simulink model "ScriptDemo"  (R2022b)
settings: configuration reference "TmVcThermal_Configuration_sub" (kept outside this file)
undefined symbols (not defined in the file): aaaa, bbbb, cTmComprCtrl_D_u8HvacFlowTable_db, cTmComprCtrl_D_u8HvacFlowTable_sw, cTmComprCtrl_n_i16ChillCmpIMax, cTmComprCtrl_n_i16ChillCmpIMin, cTmComprCtrl_n_i16ChillCmpIMin666, cTmComprCtrl_n_i16ChillCmpPMax, cTmComprCtrl_n_i16ChillCmpPMin, cTmComprCtrl_n_i16CmpChillCoolRpmKiMax, cTmComprCtrl_n_i16CmpChillCoolRpmKiMin, cTmComprCtrl_n_i16CmpChillCoolRpmKpMax, cTmComprCtrl_n_i16CmpChillCoolRpmKpMin, cTmComprCtrl_n_i16CmpCoolRpmKiMax, cTmComprCtrl_n_i16CmpCoolRpmKiMin, cTmComprCtrl_n_i16CmpCoolRpmKpMax, cTmComprCtrl_n_i16CmpCoolRpmKpMin, cTmComprCtrl_n_i16SM4CmpHeatKiMax, cTmComprCtrl_n_i16SM4CmpHeatKiMin, cTmComprCtrl_n_i16SM4CmpHeatKpMax, cTmComprCtrl_n_i16SM4CmpHeatKpMin, cTmComprCtrl_n_i16SM5CmpHeatKiMax, cTmComprCtrl_n_i16SM5CmpHeatKiMin, cTmComprCtrl_n_i16SM5CmpHeatKpMax, cTmComprCtrl_n_i16SM5CmpHeatKpMin, cTmComprCtrl_n_i16SM6CmpHeatKiMax, cTmComprCtrl_n_i16SM6CmpHeatKiMin, cTmComprCtrl_n_i16SM6CmpHeatKpMax, cTmComprCtrl_n_i16SM6CmpHeatKpMin, cTmComprCtrl_n_u16CmpMaxSpdFanFltLimt, cTmComprCtrl_n_u16CmpMaxSpdLoSidePFltLimt, cTmComprCtrl_n_u16CmpMaxSpdSensorFltLimt, cTmComprCtrl_n_u16CompMinRpm, cTmComprCtrl_n_u16CompRpmIncThres, cTmComprCtrl_t_u16BattCooltFFPeriod, cTmComprCtrl_t_u16BattCooltPIPeriod, cTmComprCtrl_t_u16CmpCoolFFPeriod, cTmComprCtrl_t_u16CmpCoolPIPeriod, cTmComprCtrl_t_u16CoolCmpChillFFPeriod, cTmComprCtrl_t_u16CoolCmpChillPIPeriod, cTmComprCtrl_t_u16SM4CmpHeatFFPeriod, cTmComprCtrl_t_u16SM4CmpHeatPIPeriod, cTmComprCtrl_t_u16SM5CmpHeatFFPeriod, cTmComprCtrl_t_u16SM5CmpHeatPIPeriod, cTmComprCtrl_t_u16SM6CmpHeatFFPeriod, cTmComprCtrl_t_u16SM6CmpHeatPIPeriod, cTmComprCtrl_Te_EvapClearInteg, cTmComprCtrl_Te_i16HpReqTempSaturoffset, cTmComprCtrl_Te_i16SatLpReplaceDiff, cTmComprCtrl_Te_i16SM3BatDiffStartEvapDecOffset, cTmComprCtrl_Te_i16SM3EvapLo, cTmComprCtrl_Te_i16SM3TBatDiffEntEvapDecOffset, cTmComprCtrl_Te_i16SM3TBatDiffEntEvapDecOffsetQuit, cTmComprCtrl_Te_s32ErrCmpChillPIContinueCoolH, cTmComprCtrl_Te_s32ErrCmpChillPIContinueCoolL, cTmComprCtrl_Te_s32ErrCmpPIContinueChillH, cTmComprCtrl_Te_s32ErrCmpPIContinueChillL, cTmComprCtrl_Te_s32ErrCmpPIContinueCoolH, cTmComprCtrl_Te_s32ErrCmpPIContinueCoolL, cTmComprCtrl_Te_s32ErrCmpPIContinueHeatH ... (+398)
libraries: simulink x782, PCMULib x640, simulink_need_slupdate x4
(part 15 of 41)

== system ScriptDemo/Create/createMerge/Before/SM6 ==
  note: 制热cycle的时候，水回路功能模式为12
  sTmSigProces_Te_s32HeatrAirTReqRamp : Inport  OutDataTypeStr=single
  sTmSigProces_Te_s32HvacHexAirTFilter : Inport  Port=2  OutDataTypeStr=single
  sTmSigProces_Te_s32TempInlet : Inport  Port=3  OutDataTypeStr=single
  sTmSigProces_Te_s32SatHp : Inport  Port=4  OutDataTypeStr=single
  sTmComprCtrl_D_u8HvacFlowLevel : Inport  Port=5  OutDataTypeStr=uint8
  xTmComprCtrl_B_CompOnReqCompOn : Inport  Port=6  OutDataTypeStr=boolean
  yTmHvchCtrl_B_HpcPtcEnad : Inport  Port=7  OutDataTypeStr=boolean
  yTmRefriModeMgr_B_HeatModeInCycle : Inport  Port=8  OutDataTypeStr=boolean
  Action Port : ActionPort
  Constant : Constant  Value=cTmComprCtrl_n_i16SM6CmpHeatKpMax  OutDataTypeStr=int16
  Constant15 : Constant  Value=cTmComprCtrl_Te_s32ErrCmpPIContinueHeatL  OutDataTypeStr=single
  Constant16 : Constant  Value=cTmComprCtrl_n_i16SM6CmpHeatKiMin  OutDataTypeStr=int16
  Constant18 : Constant  Value=cTmComprCtrl_n_i16SM6CmpHeatKiMax  OutDataTypeStr=int16
  Constant2 : Constant  Value=cTmComprCtrl_n_u16CompMinRpm
  Constant7 : Constant  Value=cTmComprCtrl_t_u16SM6CmpHeatPIPeriod  OutDataTypeStr=uint16
  Constant8 : Constant  Value=cTmComprCtrl_n_i16SM6CmpHeatKpMin  OutDataTypeStr=int16
  Constant9 : Constant  Value=cTmComprCtrl_Te_s32ErrCmpPIContinueHeatH  OutDataTypeStr=single
  ID26282_SM6FF : Subsystem
  ID26284_SM6Error : Subsystem
  Logical Operator : Logic  Operator=NOT  AllPortsSameDT=off  OutDataTypeStr=boolean
  SM6FFEnable : Subsystem
  SM6_Ki : Subsystem
  SM6_Kp : Subsystem
  rSM6_n_u16DisOverrideValue : Outport  OutDataTypeStr=uint16
  rSM6_t_u16PIPeriod : Outport  Port=2  OutDataTypeStr=uint16
  rSM6_Te_s32UpErrStop : Outport  Port=3  OutDataTypeStr=single
  rSM6_n_u16ComprRpmFF : Outport  Port=4  OutDataTypeStr=uint16
  rSM6_n_u16ComprRpmKp : Outport  Port=5  OutDataTypeStr=uint16
  rSM6_Te_s32LowErrStop : Outport  Port=6  OutDataTypeStr=single
  rSM6_n_i16KpUpLimit : Outport  Port=7  OutDataTypeStr=int16
  rSM6_n_i16KpLowLimit : Outport  Port=8  OutDataTypeStr=int16
  rSM6_n_i16KiUpLimit : Outport  Port=9  OutDataTypeStr=int16
  rSM6_n_i16KiLowLimit : Outport  Port=10  OutDataTypeStr=int16
  xSM6_B_Enable : Outport  Port=11  OutDataTypeStr=boolean
  rSM6_n_u16ComprRpmKi : Outport  Port=12  OutDataTypeStr=uint16
  rSM6_Te_s32TempError : Outport  Port=13  OutDataTypeStr=single
  wires:
  ID26284_SM6Error/1(rTmComprCtrl_Te_s32TempError) -> [rTmComprCtrl_Te_s32TempError]
  [sTmComprCtrl_D_u8HvacFlowLevel] -> ID26282_SM6FF/1(sTmComprCtrl_D_u8HvacFlowLevel)
  [sTmSigProces_Te_s32TempInlet] -> ID26282_SM6FF/2(sTmSigProces_Te_s32TempInlet)
  [sTmSigProces_Te_s32HeatrAirTReqRamp] -> ID26282_SM6FF/3(sTmSigProces_Te_s32HeatrAirTReqRamp)
  [sTmComprCtrl_D_u8HvacFlowLevel] -> SM6_Ki/1(sTmComprCtrl_D_u8HvacFlowLevel)
  [sTmSigProces_Te_s32TempInlet] -> SM6_Ki/2(sTmSigProces_Te_s32TempInlet)
  [rTmComprCtrl_Te_s32TempError] -> SM6_Ki/3(rTmComprCtrl_Te_s32TempError)
  [sTmComprCtrl_D_u8HvacFlowLevel] -> SM6_Kp/1(sTmComprCtrl_D_u8HvacFlowLevel)
  [sTmSigProces_Te_s32TempInlet] -> SM6_Kp/2(sTmSigProces_Te_s32TempInlet)
  [rTmComprCtrl_Te_s32TempError] -> SM6_Kp/3(rTmComprCtrl_Te_s32TempError)
  [sTmSigProces_Te_s32SatHp] -> ID26284_SM6Error/1(sTmSigProces_Te_s32SatHp)
  [yTmHvchCtrl_B_HpcPtcEnad] -> ID26284_SM6Error/2(yTmHvchCtrl_B_HpcPtcEnad)
  [sTmSigProces_Te_s32HeatrAirTReqRamp] -> ID26284_SM6Error/3(sTmSigProces_Te_s32HeatrAirTReqRamp)
  [sTmSigProces_Te_s32HvacHexAirTFilter] -> ID26284_SM6Error/4(sTmSigProces_Te_s32HvacHexAirTFilter)
  sTmSigProces_Te_s32HeatrAirTReqRamp/1 -> [sTmSigProces_Te_s32HeatrAirTReqRamp]
  sTmSigProces_Te_s32HvacHexAirTFilter/1 -> [sTmSigProces_Te_s32HvacHexAirTFilter]
  sTmSigProces_Te_s32TempInlet/1 -> [sTmSigProces_Te_s32TempInlet]
  sTmSigProces_Te_s32SatHp/1 -> [sTmSigProces_Te_s32SatHp]
  sTmComprCtrl_D_u8HvacFlowLevel/1 -> [sTmComprCtrl_D_u8HvacFlowLevel]
  xTmComprCtrl_B_CompOnReqCompOn/1 -> [xTmComprCtrl_B_CompOnReqCompOn]
  yTmHvchCtrl_B_HpcPtcEnad/1 -> [yTmHvchCtrl_B_HpcPtcEnad]
  ID26282_SM6FF/1(SM6FF) -> [rTmComprCtrl_n_u16ComprRpmFF]
  SM6_Ki/1(SM6Ki) -> [rTmComprCtrl_n_u16ComprRpmKi]
  SM6_Kp/1(SM6Kp) -> [rTmComprCtrl_n_u16ComprRpmKp]
  SM6FFEnable/1(SM6FFEnable_B_SM6FFEnable) -> [SM6FFEnable_B_SM6FFEnable]
  [xTmComprCtrl_B_CompOnReqCompOn] -> SM6FFEnable/1(xTmComprCtrl_B_CompOnReqCompOn)
  [SM6FFEnable_B_SM6FFEnable] -> ID26282_SM6FF/Enable
  Constant/1 -> [rTmComprCtrl_n_i16KpUpLimit]
  Constant2/1 -> [rTmComprCtrl_n_u16DisOverrideValue]
  Constant9/1 -> [rTmComprCtrl_Te_s32UpErrStop]
  Constant8/1 -> [rTmComprCtrl_n_i16KpLowLimit]
  Constant15/1 -> [rTmComprCtrl_Te_s32LowErrStop]
  Constant7/1 -> [rTmComprCtrl_t_u16PIPeriod]
  Constant16/1 -> [rTmComprCtrl_n_i16KiLowLimit]
  Logical Operator/1 -> [xTmComprCtrl_B_Enable]
  Constant18/1 -> [rTmComprCtrl_n_i16KiUpLimit]
  [yTmRefriModeMgr_B_HeatModeInCycle] -> Logical Operator/1
  yTmRefriModeMgr_B_HeatModeInCycle/1 -> [yTmRefriModeMgr_B_HeatModeInCycle]
  [rTmComprCtrl_n_u16DisOverrideValue] -> rSM6_n_u16DisOverrideValue/1
  [rTmComprCtrl_t_u16PIPeriod] -> rSM6_t_u16PIPeriod/1
  [rTmComprCtrl_Te_s32UpErrStop] -> rSM6_Te_s32UpErrStop/1
  [rTmComprCtrl_n_u16ComprRpmFF] -> rSM6_n_u16ComprRpmFF/1
  [rTmComprCtrl_n_u16ComprRpmKp] -> rSM6_n_u16ComprRpmKp/1
  [rTmComprCtrl_Te_s32LowErrStop] -> rSM6_Te_s32LowErrStop/1
  [rTmComprCtrl_n_i16KpUpLimit] -> rSM6_n_i16KpUpLimit/1
  [rTmComprCtrl_n_i16KpLowLimit] -> rSM6_n_i16KpLowLimit/1
  [rTmComprCtrl_n_i16KiUpLimit] -> rSM6_n_i16KiUpLimit/1
  [rTmComprCtrl_n_i16KiLowLimit] -> rSM6_n_i16KiLowLimit/1
  [xTmComprCtrl_B_Enable] -> xSM6_B_Enable/1
  [rTmComprCtrl_n_u16ComprRpmKi] -> rSM6_n_u16ComprRpmKi/1
  [rTmComprCtrl_Te_s32TempError] -> rSM6_Te_s32TempError/1

== system ScriptDemo/Create/createMerge/Before/SM7 ==
  sTmSigProces_Te_s32TAmb : Inport  OutDataTypeStr=single
  sTmSigProces_Te_s32HvBattCooltTOutFilter : Inport  Port=2  OutDataTypeStr=single
  Action Port : ActionPort
  2-D Lookup Table11 : Lookup_n-D  LookupTableObject=mTmComprCtrl_n_u16FFCmpSpdChillDeice  BreakpointsForDimension1=mTmComprCtrl_n_u16FFCmpSpdChillDeice_Y  BreakpointsForDimension2=mTmComprCtrl_n_u16FFCmpSpdChillDeice_X  BreakpointsForDimension1DataTypeStr=Inherit: Inherit from 'Breakpoint data'  BreakpointsForDimension2DataTypeStr=Inherit: Inherit from 'Breakpoint data'  Table=mTmComprCtrl_n_u16FFCmpSpdChillDeice  TableDataTypeStr=Inherit: Inherit from 'Table data'  ExtrapMethod=Clip  InternalRulePriority=Speed  OutDataTypeStr=Inherit: Inherit via back propagation  RndMeth=Simplest  InputSameDT=off
      settings: InputPortMap=u0,u1
  Constant : Constant  Value=0  OutDataTypeStr=uint16
  Constant1 : Constant  Value=0  OutDataTypeStr=uint16
  Constant11 : Constant  Value=5  OutDataTypeStr=uint16
  Constant12 : Constant  Value=0  OutDataTypeStr=boolean
  Constant2 : Constant  Value=0  OutDataTypeStr=uint16
  Constant3 : Constant  Value=0  OutDataTypeStr=single
  Constant4 : Constant  Value=0  OutDataTypeStr=single
  Constant5 : Constant  Value=0  OutDataTypeStr=single
  Constant{6..9} (4 alike) : Constant  Value=0  OutDataTypeStr=int16
  rSM7_n_u16DisOverrideValue : Outport  OutDataTypeStr=uint16
  rSM7_t_u16PIPeriod : Outport  Port=2  OutDataTypeStr=uint16
  xSM7_B_Enable : Outport  Port=3  OutDataTypeStr=boolean
  rSM7_n_i16KiUpLimit : Outport  Port=4  OutDataTypeStr=int16
  rSM7_n_i16KiLowLimit : Outport  Port=5  OutDataTypeStr=int16
  rSM7_Te_s32TempError : Outport  Port=6  OutDataTypeStr=single
  rSM7_n_u16ComprRpmFF : Outport  Port=7  OutDataTypeStr=uint16
  rSM7_n_u16ComprRpmKp : Outport  Port=8  OutDataTypeStr=uint16
  rSM7_n_u16ComprRpmKi : Outport  Port=9  OutDataTypeStr=uint16
  rSM7_Te_s32UpErrStop : Outport  Port=10  OutDataTypeStr=single
  rSM7_Te_s32LowErrStop : Outport  Port=11  OutDataTypeStr=single
  rSM7_n_i16KpUpLimit : Outport  Port=12  OutDataTypeStr=int16
  rSM7_n_i16KpLowLimit : Outport  Port=13  OutDataTypeStr=int16
  wires:
  [sTmSigProces_Te_s32TAmb] -> 2-D Lookup Table11/2
  [sTmSigProces_Te_s32HvBattCooltTOutFilter] -> 2-D Lookup Table11/1
  sTmSigProces_Te_s32TAmb/1 -> [sTmSigProces_Te_s32TAmb]
  sTmSigProces_Te_s32HvBattCooltTOutFilter/1 -> [sTmSigProces_Te_s32HvBattCooltTOutFilter]
  2-D Lookup Table11/1 -> [rTmComprCtrl_n_u16DisOverrideValue]
  Constant12/1 -> [xTmComprCtrl_B_Enable]
  Constant7/1 -> [rTmComprCtrl_n_i16KiUpLimit]
  Constant8/1 -> [rTmComprCtrl_n_i16KiLowLimit]
  Constant11/1 -> [rTmComprCtrl_t_u16PIPeriod]
  Constant5/1 -> [rTmComprCtrl_Te_s32LowErrStop]
  Constant/1 -> [rTmComprCtrl_n_u16ComprRpmFF]
  Constant6/1 -> [rTmComprCtrl_n_i16KpLowLimit]
  Constant1/1 -> [rTmComprCtrl_n_u16ComprRpmKp]
  Constant9/1 -> [rTmComprCtrl_n_i16KpUpLimit]
  Constant2/1 -> [rTmComprCtrl_n_u16ComprRpmKi]
  Constant4/1 -> [rTmComprCtrl_Te_s32TempError]
  Constant3/1 -> [rTmComprCtrl_Te_s32UpErrStop]
  [rTmComprCtrl_n_u16DisOverrideValue] -> rSM7_n_u16DisOverrideValue/1
  [rTmComprCtrl_t_u16PIPeriod] -> rSM7_t_u16PIPeriod/1
  [xTmComprCtrl_B_Enable] -> xSM7_B_Enable/1
  [rTmComprCtrl_n_i16KiUpLimit] -> rSM7_n_i16KiUpLimit/1
  [rTmComprCtrl_n_i16KiLowLimit] -> rSM7_n_i16KiLowLimit/1
  [rTmComprCtrl_Te_s32TempError] -> rSM7_Te_s32TempError/1
  [rTmComprCtrl_n_u16ComprRpmFF] -> rSM7_n_u16ComprRpmFF/1
  [rTmComprCtrl_n_u16ComprRpmKp] -> rSM7_n_u16ComprRpmKp/1
  [rTmComprCtrl_n_u16ComprRpmKi] -> rSM7_n_u16ComprRpmKi/1
  [rTmComprCtrl_Te_s32UpErrStop] -> rSM7_Te_s32UpErrStop/1
  [rTmComprCtrl_Te_s32LowErrStop] -> rSM7_Te_s32LowErrStop/1
  [rTmComprCtrl_n_i16KpUpLimit] -> rSM7_n_i16KpUpLimit/1
  [rTmComprCtrl_n_i16KpLowLimit] -> rSM7_n_i16KpLowLimit/1

== system ScriptDemo/Create/createPorts/createPorts/After ==
  note: % 目的: 对模型输入输出端口的信号线进行解析
      | [inCnt, outCnt,inCntDel, outCntDel] = createPorts('Template', gcs, 'sheet','Signals')
  yTmIn_B_CPSRFbSt : Inport  OutDataTypeStr=boolean
  sTmIn_D_u8CexvCalibSts : Inport  Port=2  OutDataTypeStr=uint8
  sTmDiag_D_u8EexvFltSt : Inport  Port=3  OutDataTypeStr=uint8
  sTmDiag_D_u8CexvFltSt : Inport  Port=4  OutDataTypeStr=uint8
  yTmRefriModeMgr_B_InterChillDeicing : Inport  Port=5  OutDataTypeStr=boolean
  sTmSigProces_Te_s32HeatSH : Inport  Port=6  OutDataTypeStr=single
  yTmRefriModeMgr_B_CoolOCRMode : Inport  Port=7  OutDataTypeStr=boolean
  sTmSigProces_Te_s32EvapFanReqRamp : Inport  Port=8  OutDataTypeStr=single
  sTmIn_v_s32VehSpdLgt : Inport  Port=9  OutDataTypeStr=single
  sTmSigProces_Te_s32BattHvMaxFilter : Inport  Port=10  OutDataTypeStr=single
  sTmSigProces_Te_s32EvapFanFilter : Inport  Port=11  OutDataTypeStr=single
  sTmComprCtrl_n_u16CompRpmReq : Inport  Port=12  OutDataTypeStr=uint16
  sTmComprCtrl_n_u16CompMaxRpm : Inport  Port=13  OutDataTypeStr=uint16
  sTmSigProces_Te_s32HeatrAirTReqRamp : Inport  Port=14  OutDataTypeStr=single
  sTmSigProces_md_u16BlwHeat : Inport  Port=15  OutDataTypeStr=uint16
  sTmSigProces_p_u16PHighSide : Inport  Port=16  OutDataTypeStr=uint16
  sTmSigProces_Te_s32CompDischarge : Inport  Port=17  OutDataTypeStr=single
  yTmIn_B_HmiMaxACReq : Inport  Port=18  OutDataTypeStr=boolean
  sTmSigProces_Te_s32InletCal : Inport  Port=19  OutDataTypeStr=single
  sTmSigProces_Te_s32CoolSH : Inport  Port=20  OutDataTypeStr=single
  sTmSigProces_p_u16PLowSide : Inport  Port=21  OutDataTypeStr=uint16
  sTmSigProces_md_u16BlwCool : Inport  Port=22  OutDataTypeStr=uint16
  sTmSigProces_Te_s32CurInterSC : Inport  Port=23  OutDataTypeStr=single
  yTmHvchCtrl_B_HpcPtcEnad : Inport  Port=24  OutDataTypeStr=boolean
  sTmRefriModeMgr_D_u8HpReqPTCState : Inport  Port=25  OutDataTypeStr=uint8
  yTmComprCtrl_B_CompOnReq : Inport  Port=26  OutDataTypeStr=boolean
  sTmIn_D_u8HeatPump : Inport  Port=27  OutDataTypeStr=uint8
  sTmSigProces_Te_s32HvacHexAirTFilter : Inport  Port=28  OutDataTypeStr=single
  sTmDiag_D_u8EexvPosnReq2FEnaState : Inport  Port=29  OutDataTypeStr=uint8
  sTmDiag_X_s32EexvPosnReq2F : Inport  Port=30  OutDataTypeStr=single
  sTmDiag_D_u8EexvMoveEna2FEnaState : Inport  Port=31  OutDataTypeStr=uint8
  yTmDiag_B_EexvMoveEnReq2F : Inport  Port=32  OutDataTypeStr=boolean
  sTmDiag_D_u8EexvCal2FEnaState : Inport  Port=33  OutDataTypeStr=uint8
  yTmDiag_B_EexvCalReq2F : Inport  Port=34  OutDataTypeStr=boolean
  sTmDiag_D_u8BexvPosnReq2FEnaState : Inport  Port=35  OutDataTypeStr=uint8
  sTmDiag_X_s32BexvPosnReq2F : Inport  Port=36  OutDataTypeStr=single
  sTmDiag_D_u8BexvMoveEna2FEnaState : Inport  Port=37  OutDataTypeStr=uint8
  yTmDiag_B_BexvMoveEnReq2F : Inport  Port=38  OutDataTypeStr=boolean
  sTmDiag_D_u8BexvCal2FEnaState : Inport  Port=39  OutDataTypeStr=uint8
  yTmDiag_B_BexvCalReq2F : Inport  Port=40  OutDataTypeStr=boolean
  sTmDiag_D_u8CexvPosnReq2FEnaState : Inport  Port=41  OutDataTypeStr=uint8
  sTmDiag_X_s32CexvPosnReq2F : Inport  Port=42  OutDataTypeStr=single
  sTmDiag_D_u8CexvMoveEna2FEnaState : Inport  Port=43  OutDataTypeStr=uint8
  yTmDiag_B_CexvMoveEnReq2F : Inport  Port=44  OutDataTypeStr=boolean
  sTmDiag_D_u8CexvCal2FEnaState : Inport  Port=45  OutDataTypeStr=uint8
  yTmDiag_B_CexvCalReq2F : Inport  Port=46  OutDataTypeStr=boolean
  sTmSigProces_D_u8LargerCoolingFlag : Inport  Port=47  OutDataTypeStr=uint8
  sTmComprCtrl_D_u8HvacFlowLevel : Inport  Port=48  OutDataTypeStr=uint8
  sTmRefriModeMgr_D_u8ModeSwitchType : Inport  Port=49  OutDataTypeStr=uint8
  sTmComprCtrl_D_u8CmprRefriSwitchSt : Inport  Port=50  OutDataTypeStr=uint8
  sTmIn_X_s32EexvPosSts : Inport  Port=51  OutDataTypeStr=single
  sTmIn_X_s32CexvPosSts : Inport  Port=52  OutDataTypeStr=single
  sTmIn_X_s32BexvPosSts : Inport  Port=53  OutDataTypeStr=single
  sTmSovCtrl_D_u8SOV2RefriSwitchSt : Inport  Port=54  OutDataTypeStr=uint8
  sTmDiag_D_u8EvapOutTFltSt : Inport  Port=55  OutDataTypeStr=uint8
  sTmDiag_D_u8ChillerOutTFltSt : Inport  Port=56  OutDataTypeStr=uint8
  sTmDiag_D_u8LoSidePFltSt : Inport  Port=57  OutDataTypeStr=uint8
  sTmDiag_D_u8HiSidePFltSt : Inport  Port=58  OutDataTypeStr=uint8
  sTmDiag_D_u8OutrCondOutTFltSt : Inport  Port=59  OutDataTypeStr=uint8
  sTmDiag_D_u8InrCondOutTFltSt : Inport  Port=60  OutDataTypeStr=uint8
  sTmSigProces_Pw_i16ReqPwrForCool : Inport  Port=61  OutDataTypeStr=int16
  sTmIn_L_s32HvBattCoolFlow1 : Inport  Port=62  OutDataTypeStr=single
  sTmRefriVlvCtrl_X_s32CEXVPosReq : Outport  OutDataTypeStr=single
  sTmRefriVlvCtrl_X_s32EEXVPosReq : Outport  Port=2  OutDataTypeStr=single
  sTmRefriVlvCtrl_X_s32BEXVPosReq : Outport  Port=3  OutDataTypeStr=single
  yTmRefriVlvCtrl_B_HpcCexvMovEnable : Outport  Port=4  OutDataTypeStr=boolean
  sTmRefriVlvCtrl_Z_u8CEXVInitState : Outport  Port=5  OutDataTypeStr=uint8
  yTmRefriVlvCtrl_B_CexvCalibReq : Outport  Port=6  OutDataTypeStr=boolean
  yTmRefriVlvCtrl_B_HpcEexvMovEnable : Outport  Port=7  OutDataTypeStr=boolean
  sTmRefriVlvCtrl_Z_u8EEXVInitState : Outport  Port=8  OutDataTypeStr=uint8
  yTmRefriVlvCtrl_B_EexvCalibReq : Outport  Port=9  OutDataTypeStr=boolean
  yTmRefriVlvCtrl_B_HpcBexvMovEnable : Outport  Port=10  OutDataTypeStr=boolean
  sTmRefriVlvCtrl_Z_u8BEXVInitState : Outport  Port=11  OutDataTypeStr=uint8
  yTmRefriVlvCtrl_B_BexvCalibReq : Outport  Port=12  OutDataTypeStr=boolean
  sTmRefriVlvCtrl_X_s32SM3BexvMaxPos : Outport  Port=13  OutDataTypeStr=single
  yTmRefriVlvCtrl_B_EvapBattTLimBexvEna : Outport  Port=14  OutDataTypeStr=boolean
  sTmRefriVlvCtrl_D_u8EexvRefriSwitchSt : Outport  Port=15  OutDataTypeStr=uint8
  sTmRefriVlvCtrl_D_u8CexvRefriSwitchSt : Outport  Port=16  OutDataTypeStr=uint8
  sTmRefriVlvCtrl_D_u8BexvRefriSwitchSt : Outport  Port=17  OutDataTypeStr=uint8

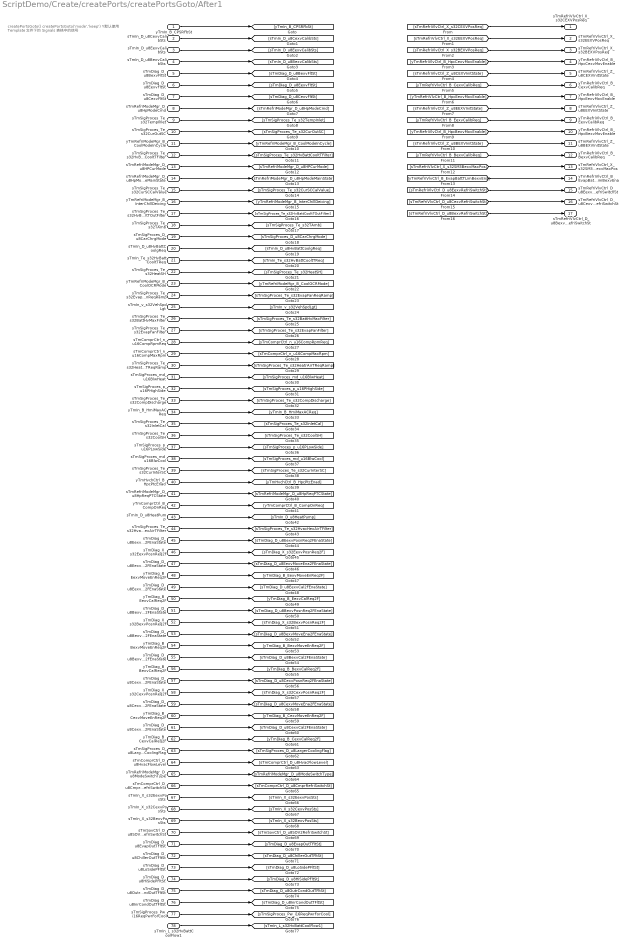
== system ScriptDemo/Create/createPorts/createPortsGoto/After1 ==
  note: createPortsGoto()
      | createPortsGoto('mode','keep')
      | % 默认使用 Template 文件下的 Signals 表格中的信号
  yTmIn_B_CPSRFbSt : Inport  OutDataTypeStr=boolean
  sTmIn_D_u8CexvCalibSts : Inport  Port=2  OutDataTypeStr=uint8
  sTmIn_D_u8EexvCalibSts : Inport  Port=3  OutDataTypeStr=uint8
  sTmIn_D_u8BexvCalibSts : Inport  Port=4  OutDataTypeStr=uint8
  sTmDiag_D_u8BexvFltSt : Inport  Port=5  OutDataTypeStr=uint8
  sTmDiag_D_u8EexvFltSt : Inport  Port=6  OutDataTypeStr=uint8
  sTmDiag_D_u8CexvFltSt : Inport  Port=7  OutDataTypeStr=uint8
  sTmRefriModeMgr_D_u8HpModeCmd : Inport  Port=8  OutDataTypeStr=uint8
  sTmSigProces_Te_s32TempInlet : Inport  Port=9  OutDataTypeStr=single
  sTmSigProces_Te_s32CurOutSC : Inport  Port=10  OutDataTypeStr=single
  yTmRefriModeMgr_B_CoolModeInCycle : Inport  Port=11  OutDataTypeStr=boolean
  sTmSigProces_Te_s32HvBattCooltTFilter : Inport  Port=12  OutDataTypeStr=single
  sTmRefriModeMgr_D_u8HPCurMode : Inport  Port=13  OutDataTypeStr=uint8
  sTmRefriModeMgr_D_u8HpModeMainState : Inport  Port=14  OutDataTypeStr=uint8
  sTmSigProces_Te_s32CurSCCalValue : Inport  Port=15  OutDataTypeStr=single
  yTmRefriModeMgr_B_InterChillDeicing : Inport  Port=16  OutDataTypeStr=boolean
  sTmSigProces_Te_s32HvBattCooltTOutFilter : Inport  Port=17  OutDataTypeStr=single
  sTmSigProces_Te_s32TAmb : Inport  Port=18  OutDataTypeStr=single
  sTmSigProces_D_u8CarChrgMode : Inport  Port=19  OutDataTypeStr=uint8
  sTmIn_D_u8HvBattCoolgReq : Inport  Port=20  OutDataTypeStr=uint8
  sTmIn_Te_s32HvBattCooltTReq : Inport  Port=21  OutDataTypeStr=single
  sTmSigProces_Te_s32HeatSH : Inport  Port=22  OutDataTypeStr=single
  yTmRefriModeMgr_B_CoolOCRMode : Inport  Port=23  OutDataTypeStr=boolean
  sTmSigProces_Te_s32EvapFanReqRamp : Inport  Port=24  OutDataTypeStr=single
  sTmIn_v_s32VehSpdLgt : Inport  Port=25  OutDataTypeStr=single
  sTmSigProces_Te_s32BattHvMaxFilter : Inport  Port=26  OutDataTypeStr=single
  sTmSigProces_Te_s32EvapFanFilter : Inport  Port=27  OutDataTypeStr=single
  sTmComprCtrl_n_u16CompRpmReq : Inport  Port=28  OutDataTypeStr=uint16
  sTmComprCtrl_n_u16CompMaxRpm : Inport  Port=29  OutDataTypeStr=uint16
  sTmSigProces_Te_s32HeatrAirTReqRamp : Inport  Port=30  OutDataTypeStr=single
  sTmSigProces_md_u16BlwHeat : Inport  Port=31  OutDataTypeStr=uint16
  sTmSigProces_p_u16PHighSide : Inport  Port=32  OutDataTypeStr=uint16
  sTmSigProces_Te_s32CompDischarge : Inport  Port=33  OutDataTypeStr=single
  yTmIn_B_HmiMaxACReq : Inport  Port=34  OutDataTypeStr=boolean
  sTmSigProces_Te_s32InletCal : Inport  Port=35  OutDataTypeStr=single
  sTmSigProces_Te_s32CoolSH : Inport  Port=36  OutDataTypeStr=single
  sTmSigProces_p_u16PLowSide : Inport  Port=37  OutDataTypeStr=uint16
  sTmSigProces_md_u16BlwCool : Inport  Port=38  OutDataTypeStr=uint16
  sTmSigProces_Te_s32CurInterSC : Inport  Port=39  OutDataTypeStr=single
  yTmHvchCtrl_B_HpcPtcEnad : Inport  Port=40  OutDataTypeStr=boolean
  sTmRefriModeMgr_D_u8HpReqPTCState : Inport  Port=41  OutDataTypeStr=uint8
  yTmComprCtrl_B_CompOnReq : Inport  Port=42  OutDataTypeStr=boolean
  sTmIn_D_u8HeatPump : Inport  Port=43  OutDataTypeStr=uint8
  sTmSigProces_Te_s32HvacHexAirTFilter : Inport  Port=44  OutDataTypeStr=single
  sTmDiag_D_u8EexvPosnReq2FEnaState : Inport  Port=45  OutDataTypeStr=uint8
  sTmDiag_X_s32EexvPosnReq2F : Inport  Port=46  OutDataTypeStr=single
  sTmDiag_D_u8EexvMoveEna2FEnaState : Inport  Port=47  OutDataTypeStr=uint8
  yTmDiag_B_EexvMoveEnReq2F : Inport  Port=48  OutDataTypeStr=boolean
  sTmDiag_D_u8EexvCal2FEnaState : Inport  Port=49  OutDataTypeStr=uint8
  yTmDiag_B_EexvCalReq2F : Inport  Port=50  OutDataTypeStr=boolean
  sTmDiag_D_u8BexvPosnReq2FEnaState : Inport  Port=51  OutDataTypeStr=uint8
  sTmDiag_X_s32BexvPosnReq2F : Inport  Port=52  OutDataTypeStr=single
  sTmDiag_D_u8BexvMoveEna2FEnaState : Inport  Port=53  OutDataTypeStr=uint8
  yTmDiag_B_BexvMoveEnReq2F : Inport  Port=54  OutDataTypeStr=boolean
  sTmDiag_D_u8BexvCal2FEnaState : Inport  Port=55  OutDataTypeStr=uint8
  yTmDiag_B_BexvCalReq2F : Inport  Port=56  OutDataTypeStr=boolean
  sTmDiag_D_u8CexvPosnReq2FEnaState : Inport  Port=57  OutDataTypeStr=uint8
  sTmDiag_X_s32CexvPosnReq2F : Inport  Port=58  OutDataTypeStr=single
  sTmDiag_D_u8CexvMoveEna2FEnaState : Inport  Port=59  OutDataTypeStr=uint8
  yTmDiag_B_CexvMoveEnReq2F : Inport  Port=60  OutDataTypeStr=boolean
  sTmDiag_D_u8CexvCal2FEnaState : Inport  Port=61  OutDataTypeStr=uint8
  yTmDiag_B_CexvCalReq2F : Inport  Port=62  OutDataTypeStr=boolean
  sTmSigProces_D_u8LargerCoolingFlag : Inport  Port=63  OutDataTypeStr=uint8
  sTmComprCtrl_D_u8HvacFlowLevel : Inport  Port=64  OutDataTypeStr=uint8
  sTmRefriModeMgr_D_u8ModeSwitchType : Inport  Port=65  OutDataTypeStr=uint8
  sTmComprCtrl_D_u8CmprRefriSwitchSt : Inport  Port=66  OutDataTypeStr=uint8
  sTmIn_X_s32EexvPosSts : Inport  Port=67  OutDataTypeStr=single
  sTmIn_X_s32CexvPosSts : Inport  Port=68  OutDataTypeStr=single
  sTmIn_X_s32BexvPosSts : Inport  Port=69  OutDataTypeStr=single
  sTmSovCtrl_D_u8SOV2RefriSwitchSt : Inport  Port=70  OutDataTypeStr=uint8
  sTmDiag_D_u8EvapOutTFltSt : Inport  Port=71  OutDataTypeStr=uint8
  sTmDiag_D_u8ChillerOutTFltSt : Inport  Port=72  OutDataTypeStr=uint8
  sTmDiag_D_u8LoSidePFltSt : Inport  Port=73  OutDataTypeStr=uint8
  sTmDiag_D_u8HiSidePFltSt : Inport  Port=74  OutDataTypeStr=uint8
  sTmDiag_D_u8OutrCondOutTFltSt : Inport  Port=75  OutDataTypeStr=uint8
  sTmDiag_D_u8InrCondOutTFltSt : Inport  Port=76  OutDataTypeStr=uint8
  sTmSigProces_Pw_i16ReqPwrForCool : Inport  Port=77  OutDataTypeStr=int16
  sTmIn_L_s32HvBattCoolFlow1 : Inport  Port=78  OutDataTypeStr=single
  sTmRefriVlvCtrl_X_s32CEXVPosReq : Outport  OutDataTypeStr=single
  sTmRefriVlvCtrl_X_s32EEXVPosReq : Outport  Port=2  OutDataTypeStr=single
  sTmRefriVlvCtrl_X_s32BEXVPosReq : Outport  Port=3  OutDataTypeStr=single
  yTmRefriVlvCtrl_B_HpcCexvMovEnable : Outport  Port=4  OutDataTypeStr=boolean
  sTmRefriVlvCtrl_Z_u8CEXVInitState : Outport  Port=5  OutDataTypeStr=uint8
  yTmRefriVlvCtrl_B_CexvCalibReq : Outport  Port=6  OutDataTypeStr=boolean
  yTmRefriVlvCtrl_B_HpcEexvMovEnable : Outport  Port=7  OutDataTypeStr=boolean
  sTmRefriVlvCtrl_Z_u8EEXVInitState : Outport  Port=8  OutDataTypeStr=uint8
  yTmRefriVlvCtrl_B_EexvCalibReq : Outport  Port=9  OutDataTypeStr=boolean
  yTmRefriVlvCtrl_B_HpcBexvMovEnable : Outport  Port=10  OutDataTypeStr=boolean
  sTmRefriVlvCtrl_Z_u8BEXVInitState : Outport  Port=11  OutDataTypeStr=uint8
  yTmRefriVlvCtrl_B_BexvCalibReq : Outport  Port=12  OutDataTypeStr=boolean
  sTmRefriVlvCtrl_X_s32SM3BexvMaxPos : Outport  Port=13  OutDataTypeStr=single
  yTmRefriVlvCtrl_B_EvapBattTLimBexvEna : Outport  Port=14  OutDataTypeStr=boolean
  sTmRefriVlvCtrl_D_u8EexvRefriSwitchSt : Outport  Port=15  OutDataTypeStr=uint8
  sTmRefriVlvCtrl_D_u8CexvRefriSwitchSt : Outport  Port=16  OutDataTypeStr=uint8
  sTmRefriVlvCtrl_D_u8BexvRefriSwitchSt : Outport  Port=17  OutDataTypeStr=uint8
  wires:
  sTmDiag_D_u8EvapOutTFltSt/1 -> [sTmDiag_D_u8EvapOutTFltSt]
  [yTmRefriVlvCtrl_B_HpcBexvMovEnable] -> yTmRefriVlvCtrl_B_HpcBexvMovEnable/1
  sTmRefriModeMgr_D_u8HpReqPTCState/1 -> [sTmRefriModeMgr_D_u8HpReqPTCState]
  [yTmRefriVlvCtrl_B_EvapBattTLimBexvEna] -> yTmRefriVlvCtrl_B_EvapBattTLimBexvEna/1
  sTmSigProces_Te_s32CompDischarge/1 -> [sTmSigProces_Te_s32CompDischarge]
  [sTmRefriVlvCtrl_Z_u8CEXVInitState] -> sTmRefriVlvCtrl_Z_u8CEXVInitState/1
  sTmSigProces_md_u16BlwHeat/1 -> [sTmSigProces_md_u16BlwHeat]
  [yTmRefriVlvCtrl_B_EexvCalibReq] -> yTmRefriVlvCtrl_B_EexvCalibReq/1
  sTmDiag_D_u8EexvCal2FEnaState/1 -> [sTmDiag_D_u8EexvCal2FEnaState]
  [sTmRefriVlvCtrl_X_s32BEXVPosReq] -> sTmRefriVlvCtrl_X_s32BEXVPosReq/1
  [sTmRefriVlvCtrl_Z_u8BEXVInitState] -> sTmRefriVlvCtrl_Z_u8BEXVInitState/1
  [sTmRefriVlvCtrl_X_s32EEXVPosReq] -> sTmRefriVlvCtrl_X_s32EEXVPosReq/1
  yTmRefriModeMgr_B_CoolModeInCycle/1 -> [yTmRefriModeMgr_B_CoolModeInCycle]
  sTmSigProces_Te_s32HvBattCooltTOutFilter/1 -> [sTmSigProces_Te_s32HvBattCooltTOutFilter]
  yTmDiag_B_EexvMoveEnReq2F/1 -> [yTmDiag_B_EexvMoveEnReq2F]
  sTmDiag_D_u8OutrCondOutTFltSt/1 -> [sTmDiag_D_u8OutrCondOutTFltSt]
  sTmDiag_D_u8EexvMoveEna2FEnaState/1 -> [sTmDiag_D_u8EexvMoveEna2FEnaState]
  sTmSigProces_Te_s32CurInterSC/1 -> [sTmSigProces_Te_s32CurInterSC]
  sTmSigProces_Te_s32BattHvMaxFilter/1 -> [sTmSigProces_Te_s32BattHvMaxFilter]
  yTmHvchCtrl_B_HpcPtcEnad/1 -> [yTmHvchCtrl_B_HpcPtcEnad]
  sTmIn_D_u8HeatPump/1 -> [sTmIn_D_u8HeatPump]
  sTmComprCtrl_n_u16CompMaxRpm/1 -> [sTmComprCtrl_n_u16CompMaxRpm]
  [sTmRefriVlvCtrl_X_s32SM3BexvMaxPos] -> sTmRefriVlvCtrl_X_s32SM3BexvMaxPos/1
  yTmComprCtrl_B_CompOnReq/1 -> [yTmComprCtrl_B_CompOnReq]
  sTmSigProces_Te_s32HvacHexAirTFilter/1 -> [sTmSigProces_Te_s32HvacHexAirTFilter]
  sTmIn_D_u8CexvCalibSts/1 -> [sTmIn_D_u8CexvCalibSts]
  sTmComprCtrl_D_u8CmprRefriSwitchSt/1 -> [sTmComprCtrl_D_u8CmprRefriSwitchSt]
  sTmIn_D_u8HvBattCoolgReq/1 -> [sTmIn_D_u8HvBattCoolgReq]
  sTmDiag_D_u8EexvPosnReq2FEnaState/1 -> [sTmDiag_D_u8EexvPosnReq2FEnaState]
  sTmSigProces_D_u8CarChrgMode/1 -> [sTmSigProces_D_u8CarChrgMode]
  yTmRefriModeMgr_B_CoolOCRMode/1 -> [yTmRefriModeMgr_B_CoolOCRMode]
  sTmIn_L_s32HvBattCoolFlow1/1 -> [sTmIn_L_s32HvBattCoolFlow1]
  sTmDiag_X_s32BexvPosnReq2F/1 -> [sTmDiag_X_s32BexvPosnReq2F]
  sTmDiag_X_s32EexvPosnReq2F/1 -> [sTmDiag_X_s32EexvPosnReq2F]
  yTmDiag_B_EexvCalReq2F/1 -> [yTmDiag_B_EexvCalReq2F]
  sTmDiag_D_u8LoSidePFltSt/1 -> [sTmDiag_D_u8LoSidePFltSt]
  sTmSigProces_Te_s32EvapFanFilter/1 -> [sTmSigProces_Te_s32EvapFanFilter]
  sTmSigProces_Te_s32HeatSH/1 -> [sTmSigProces_Te_s32HeatSH]
  sTmComprCtrl_n_u16CompRpmReq/1 -> [sTmComprCtrl_n_u16CompRpmReq]
  sTmRefriModeMgr_D_u8HpModeMainState/1 -> [sTmRefriModeMgr_D_u8HpModeMainState]
  sTmSigProces_Te_s32CurSCCalValue/1 -> [sTmSigProces_Te_s32CurSCCalValue]
  yTmIn_B_HmiMaxACReq/1 -> [yTmIn_B_HmiMaxACReq]
  yTmRefriModeMgr_B_InterChillDeicing/1 -> [yTmRefriModeMgr_B_InterChillDeicing]
  sTmSigProces_Te_s32HeatrAirTReqRamp/1 -> [sTmSigProces_Te_s32HeatrAirTReqRamp]
  [sTmRefriVlvCtrl_X_s32CEXVPosReq] -> sTmRefriVlvCtrl_X_s32CEXVPosReq/1
  sTmSigProces_Te_s32InletCal/1 -> [sTmSigProces_Te_s32InletCal]
  sTmSigProces_p_u16PHighSide/1 -> [sTmSigProces_p_u16PHighSide]
  sTmIn_Te_s32HvBattCooltTReq/1 -> [sTmIn_Te_s32HvBattCooltTReq]
  [yTmRefriVlvCtrl_B_BexvCalibReq] -> yTmRefriVlvCtrl_B_BexvCalibReq/1
  sTmSigProces_Te_s32CoolSH/1 -> [sTmSigProces_Te_s32CoolSH]
  sTmSigProces_p_u16PLowSide/1 -> [sTmSigProces_p_u16PLowSide]
  [sTmRefriVlvCtrl_Z_u8EEXVInitState] -> sTmRefriVlvCtrl_Z_u8EEXVInitState/1
  sTmDiag_D_u8HiSidePFltSt/1 -> [sTmDiag_D_u8HiSidePFltSt]
  [yTmRefriVlvCtrl_B_HpcEexvMovEnable] -> yTmRefriVlvCtrl_B_HpcEexvMovEnable/1
  sTmSigProces_md_u16BlwCool/1 -> [sTmSigProces_md_u16BlwCool]
  sTmDiag_D_u8ChillerOutTFltSt/1 -> [sTmDiag_D_u8ChillerOutTFltSt]
  sTmSigProces_Te_s32TAmb/1 -> [sTmSigProces_Te_s32TAmb]
  sTmDiag_D_u8InrCondOutTFltSt/1 -> [sTmDiag_D_u8InrCondOutTFltSt]
  [sTmRefriVlvCtrl_D_u8EexvRefriSwitchSt] -> sTmRefriVlvCtrl_D_u8EexvRefriSwitchSt/1
  [yTmRefriVlvCtrl_B_CexvCalibReq] -> yTmRefriVlvCtrl_B_CexvCalibReq/1
  sTmSigProces_Te_s32EvapFanReqRamp/1 -> [sTmSigProces_Te_s32EvapFanReqRamp]
  [yTmRefriVlvCtrl_B_HpcCexvMovEnable] -> yTmRefriVlvCtrl_B_HpcCexvMovEnable/1
  yTmIn_B_CPSRFbSt/1 -> [yTmIn_B_CPSRFbSt]
  sTmSigProces_Pw_i16ReqPwrForCool/1 -> [sTmSigProces_Pw_i16ReqPwrForCool]
  sTmIn_v_s32VehSpdLgt/1 -> [sTmIn_v_s32VehSpdLgt]
  sTmIn_D_u8EexvCalibSts/1 -> [sTmIn_D_u8EexvCalibSts]
  sTmDiag_D_u8BexvFltSt/1 -> [sTmDiag_D_u8BexvFltSt]
  sTmIn_D_u8BexvCalibSts/1 -> [sTmIn_D_u8BexvCalibSts]
  sTmDiag_D_u8EexvFltSt/1 -> [sTmDiag_D_u8EexvFltSt]
  sTmDiag_D_u8CexvFltSt/1 -> [sTmDiag_D_u8CexvFltSt]
  sTmSigProces_Te_s32TempInlet/1 -> [sTmSigProces_Te_s32TempInlet]
  sTmRefriModeMgr_D_u8HpModeCmd/1 -> [sTmRefriModeMgr_D_u8HpModeCmd]
  sTmSigProces_Te_s32CurOutSC/1 -> [sTmSigProces_Te_s32CurOutSC]
  sTmSigProces_Te_s32HvBattCooltTFilter/1 -> [sTmSigProces_Te_s32HvBattCooltTFilter]
  sTmRefriModeMgr_D_u8HPCurMode/1 -> [sTmRefriModeMgr_D_u8HPCurMode]
  sTmDiag_D_u8BexvPosnReq2FEnaState/1 -> [sTmDiag_D_u8BexvPosnReq2FEnaState]
  sTmDiag_D_u8BexvMoveEna2FEnaState/1 -> [sTmDiag_D_u8BexvMoveEna2FEnaState]
  yTmDiag_B_BexvMoveEnReq2F/1 -> [yTmDiag_B_BexvMoveEnReq2F]
  sTmDiag_D_u8BexvCal2FEnaState/1 -> [sTmDiag_D_u8BexvCal2FEnaState]
  yTmDiag_B_BexvCalReq2F/1 -> [yTmDiag_B_BexvCalReq2F]
  sTmDiag_D_u8CexvPosnReq2FEnaState/1 -> [sTmDiag_D_u8CexvPosnReq2FEnaState]
  sTmDiag_X_s32CexvPosnReq2F/1 -> [sTmDiag_X_s32CexvPosnReq2F]
  sTmDiag_D_u8CexvMoveEna2FEnaState/1 -> [sTmDiag_D_u8CexvMoveEna2FEnaState]
  yTmDiag_B_CexvMoveEnReq2F/1 -> [yTmDiag_B_CexvMoveEnReq2F]
  sTmDiag_D_u8CexvCal2FEnaState/1 -> [sTmDiag_D_u8CexvCal2FEnaState]
  yTmDiag_B_CexvCalReq2F/1 -> [yTmDiag_B_CexvCalReq2F]
  sTmComprCtrl_D_u8HvacFlowLevel/1 -> [sTmComprCtrl_D_u8HvacFlowLevel]
  sTmRefriModeMgr_D_u8ModeSwitchType/1 -> [sTmRefriModeMgr_D_u8ModeSwitchType]
  sTmSigProces_D_u8LargerCoolingFlag/1 -> [sTmSigProces_D_u8LargerCoolingFlag]
  sTmIn_X_s32EexvPosSts/1 -> [sTmIn_X_s32EexvPosSts]
  sTmIn_X_s32CexvPosSts/1 -> [sTmIn_X_s32CexvPosSts]
  sTmIn_X_s32BexvPosSts/1 -> [sTmIn_X_s32BexvPosSts]
  sTmSovCtrl_D_u8SOV2RefriSwitchSt/1 -> [sTmSovCtrl_D_u8SOV2RefriSwitchSt]
  [sTmRefriVlvCtrl_D_u8CexvRefriSwitchSt] -> sTmRefriVlvCtrl_D_u8CexvRefriSwitchSt/1
  [sTmRefriVlvCtrl_D_u8BexvRefriSwitchSt] -> sTmRefriVlvCtrl_D_u8BexvRefriSwitchSt/1

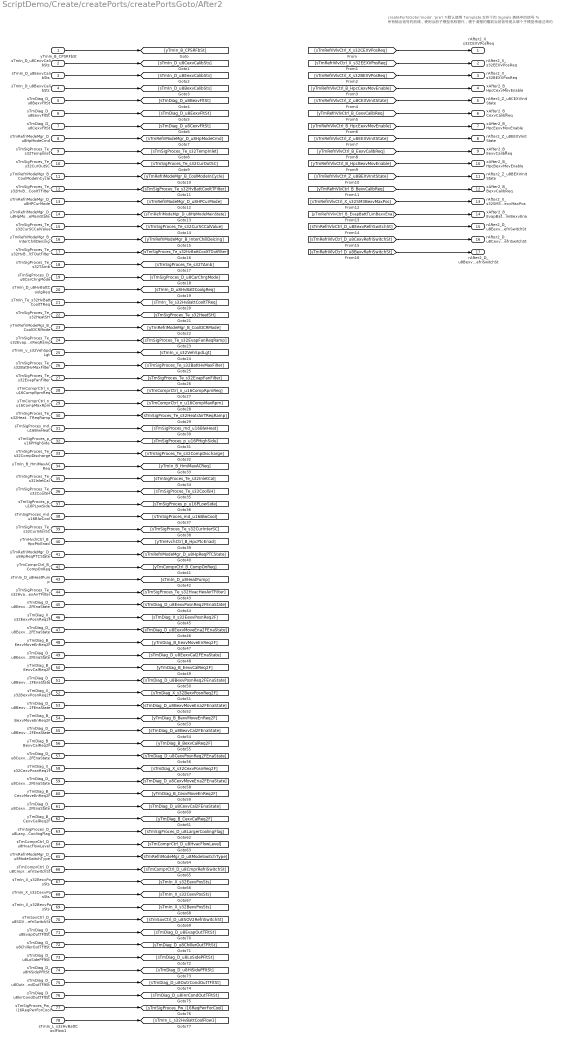
== system ScriptDemo/Create/createPorts/createPortsGoto/After2 ==
  note: createPortsGoto('mode','pre')
      | % 默认使用 Template 文件下的 Signals 表格中的信号
      | % 所有输出信号的前缀，使用当前子模型名称替代，便于清楚的看到当前信号是从哪个子模型传递过来的
  yTmIn_B_CPSRFbSt : Inport  OutDataTypeStr=boolean
  sTmIn_D_u8CexvCalibSts : Inport  Port=2  OutDataTypeStr=uint8
  sTmIn_D_u8EexvCalibSts : Inport  Port=3  OutDataTypeStr=uint8
  sTmIn_D_u8BexvCalibSts : Inport  Port=4  OutDataTypeStr=uint8
  sTmDiag_D_u8BexvFltSt : Inport  Port=5  OutDataTypeStr=uint8
  sTmDiag_D_u8EexvFltSt : Inport  Port=6  OutDataTypeStr=uint8
  sTmDiag_D_u8CexvFltSt : Inport  Port=7  OutDataTypeStr=uint8
  sTmRefriModeMgr_D_u8HpModeCmd : Inport  Port=8  OutDataTypeStr=uint8
  sTmSigProces_Te_s32TempInlet : Inport  Port=9  OutDataTypeStr=single
  sTmSigProces_Te_s32CurOutSC : Inport  Port=10  OutDataTypeStr=single
  yTmRefriModeMgr_B_CoolModeInCycle : Inport  Port=11  OutDataTypeStr=boolean
  sTmSigProces_Te_s32HvBattCooltTFilter : Inport  Port=12  OutDataTypeStr=single
  sTmRefriModeMgr_D_u8HPCurMode : Inport  Port=13  OutDataTypeStr=uint8
  sTmRefriModeMgr_D_u8HpModeMainState : Inport  Port=14  OutDataTypeStr=uint8
  sTmSigProces_Te_s32CurSCCalValue : Inport  Port=15  OutDataTypeStr=single
  yTmRefriModeMgr_B_InterChillDeicing : Inport  Port=16  OutDataTypeStr=boolean
  sTmSigProces_Te_s32HvBattCooltTOutFilter : Inport  Port=17  OutDataTypeStr=single
  sTmSigProces_Te_s32TAmb : Inport  Port=18  OutDataTypeStr=single
  sTmSigProces_D_u8CarChrgMode : Inport  Port=19  OutDataTypeStr=uint8
  sTmIn_D_u8HvBattCoolgReq : Inport  Port=20  OutDataTypeStr=uint8
  sTmIn_Te_s32HvBattCooltTReq : Inport  Port=21  OutDataTypeStr=single
  sTmSigProces_Te_s32HeatSH : Inport  Port=22  OutDataTypeStr=single
  yTmRefriModeMgr_B_CoolOCRMode : Inport  Port=23  OutDataTypeStr=boolean
  sTmSigProces_Te_s32EvapFanReqRamp : Inport  Port=24  OutDataTypeStr=single
  sTmIn_v_s32VehSpdLgt : Inport  Port=25  OutDataTypeStr=single
  sTmSigProces_Te_s32BattHvMaxFilter : Inport  Port=26  OutDataTypeStr=single
  sTmSigProces_Te_s32EvapFanFilter : Inport  Port=27  OutDataTypeStr=single
  sTmComprCtrl_n_u16CompRpmReq : Inport  Port=28  OutDataTypeStr=uint16
  sTmComprCtrl_n_u16CompMaxRpm : Inport  Port=29  OutDataTypeStr=uint16
  sTmSigProces_Te_s32HeatrAirTReqRamp : Inport  Port=30  OutDataTypeStr=single
  sTmSigProces_md_u16BlwHeat : Inport  Port=31  OutDataTypeStr=uint16
  sTmSigProces_p_u16PHighSide : Inport  Port=32  OutDataTypeStr=uint16
  sTmSigProces_Te_s32CompDischarge : Inport  Port=33  OutDataTypeStr=single
  yTmIn_B_HmiMaxACReq : Inport  Port=34  OutDataTypeStr=boolean
  sTmSigProces_Te_s32InletCal : Inport  Port=35  OutDataTypeStr=single
  sTmSigProces_Te_s32CoolSH : Inport  Port=36  OutDataTypeStr=single
  sTmSigProces_p_u16PLowSide : Inport  Port=37  OutDataTypeStr=uint16
  sTmSigProces_md_u16BlwCool : Inport  Port=38  OutDataTypeStr=uint16
  sTmSigProces_Te_s32CurInterSC : Inport  Port=39  OutDataTypeStr=single
  yTmHvchCtrl_B_HpcPtcEnad : Inport  Port=40  OutDataTypeStr=boolean
  sTmRefriModeMgr_D_u8HpReqPTCState : Inport  Port=41  OutDataTypeStr=uint8
  yTmComprCtrl_B_CompOnReq : Inport  Port=42  OutDataTypeStr=boolean
  sTmIn_D_u8HeatPump : Inport  Port=43  OutDataTypeStr=uint8
  sTmSigProces_Te_s32HvacHexAirTFilter : Inport  Port=44  OutDataTypeStr=single
  sTmDiag_D_u8EexvPosnReq2FEnaState : Inport  Port=45  OutDataTypeStr=uint8
  sTmDiag_X_s32EexvPosnReq2F : Inport  Port=46  OutDataTypeStr=single
  sTmDiag_D_u8EexvMoveEna2FEnaState : Inport  Port=47  OutDataTypeStr=uint8
  yTmDiag_B_EexvMoveEnReq2F : Inport  Port=48  OutDataTypeStr=boolean
  sTmDiag_D_u8EexvCal2FEnaState : Inport  Port=49  OutDataTypeStr=uint8
  yTmDiag_B_EexvCalReq2F : Inport  Port=50  OutDataTypeStr=boolean
  sTmDiag_D_u8BexvPosnReq2FEnaState : Inport  Port=51  OutDataTypeStr=uint8
  sTmDiag_X_s32BexvPosnReq2F : Inport  Port=52  OutDataTypeStr=single
  sTmDiag_D_u8BexvMoveEna2FEnaState : Inport  Port=53  OutDataTypeStr=uint8
  yTmDiag_B_BexvMoveEnReq2F : Inport  Port=54  OutDataTypeStr=boolean
  sTmDiag_D_u8BexvCal2FEnaState : Inport  Port=55  OutDataTypeStr=uint8
  yTmDiag_B_BexvCalReq2F : Inport  Port=56  OutDataTypeStr=boolean
  sTmDiag_D_u8CexvPosnReq2FEnaState : Inport  Port=57  OutDataTypeStr=uint8
  sTmDiag_X_s32CexvPosnReq2F : Inport  Port=58  OutDataTypeStr=single
  sTmDiag_D_u8CexvMoveEna2FEnaState : Inport  Port=59  OutDataTypeStr=uint8
  yTmDiag_B_CexvMoveEnReq2F : Inport  Port=60  OutDataTypeStr=boolean
  sTmDiag_D_u8CexvCal2FEnaState : Inport  Port=61  OutDataTypeStr=uint8
  yTmDiag_B_CexvCalReq2F : Inport  Port=62  OutDataTypeStr=boolean
  sTmSigProces_D_u8LargerCoolingFlag : Inport  Port=63  OutDataTypeStr=uint8
  sTmComprCtrl_D_u8HvacFlowLevel : Inport  Port=64  OutDataTypeStr=uint8
  sTmRefriModeMgr_D_u8ModeSwitchType : Inport  Port=65  OutDataTypeStr=uint8
  sTmComprCtrl_D_u8CmprRefriSwitchSt : Inport  Port=66  OutDataTypeStr=uint8
  sTmIn_X_s32EexvPosSts : Inport  Port=67  OutDataTypeStr=single
  sTmIn_X_s32CexvPosSts : Inport  Port=68  OutDataTypeStr=single
  sTmIn_X_s32BexvPosSts : Inport  Port=69  OutDataTypeStr=single
  sTmSovCtrl_D_u8SOV2RefriSwitchSt : Inport  Port=70  OutDataTypeStr=uint8
  sTmDiag_D_u8EvapOutTFltSt : Inport  Port=71  OutDataTypeStr=uint8
  sTmDiag_D_u8ChillerOutTFltSt : Inport  Port=72  OutDataTypeStr=uint8
  sTmDiag_D_u8LoSidePFltSt : Inport  Port=73  OutDataTypeStr=uint8
  sTmDiag_D_u8HiSidePFltSt : Inport  Port=74  OutDataTypeStr=uint8
  sTmDiag_D_u8OutrCondOutTFltSt : Inport  Port=75  OutDataTypeStr=uint8
  sTmDiag_D_u8InrCondOutTFltSt : Inport  Port=76  OutDataTypeStr=uint8
  sTmSigProces_Pw_i16ReqPwrForCool : Inport  Port=77  OutDataTypeStr=int16
  sTmIn_L_s32HvBattCoolFlow1 : Inport  Port=78  OutDataTypeStr=single
  rAfter2_X_s32CEXVPosReq : Outport  OutDataTypeStr=single
  rAfter2_X_s32EEXVPosReq : Outport  Port=2  OutDataTypeStr=single
  rAfter2_X_s32BEXVPosReq : Outport  Port=3  OutDataTypeStr=single
  xAfter2_B_HpcCexvMovEnable : Outport  Port=4  OutDataTypeStr=boolean
  rAfter2_Z_u8CEXVInitState : Outport  Port=5  OutDataTypeStr=uint8
  xAfter2_B_CexvCalibReq : Outport  Port=6  OutDataTypeStr=boolean
  xAfter2_B_HpcEexvMovEnable : Outport  Port=7  OutDataTypeStr=boolean
  rAfter2_Z_u8EEXVInitState : Outport  Port=8  OutDataTypeStr=uint8
  xAfter2_B_EexvCalibReq : Outport  Port=9  OutDataTypeStr=boolean
  xAfter2_B_HpcBexvMovEnable : Outport  Port=10  OutDataTypeStr=boolean
  rAfter2_Z_u8BEXVInitState : Outport  Port=11  OutDataTypeStr=uint8
  xAfter2_B_BexvCalibReq : Outport  Port=12  OutDataTypeStr=boolean
  rAfter2_X_s32SM3BexvMaxPos : Outport  Port=13  OutDataTypeStr=single
  xAfter2_B_EvapBattTLimBexvEna : Outport  Port=14  OutDataTypeStr=boolean
  rAfter2_D_u8EexvRefriSwitchSt : Outport  Port=15  OutDataTypeStr=uint8
  rAfter2_D_u8CexvRefriSwitchSt : Outport  Port=16  OutDataTypeStr=uint8
  rAfter2_D_u8BexvRefriSwitchSt : Outport  Port=17  OutDataTypeStr=uint8
  wires:
  yTmIn_B_CPSRFbSt/1 -> [yTmIn_B_CPSRFbSt]
  sTmIn_D_u8CexvCalibSts/1 -> [sTmIn_D_u8CexvCalibSts]
  sTmIn_D_u8EexvCalibSts/1 -> [sTmIn_D_u8EexvCalibSts]
  sTmIn_D_u8BexvCalibSts/1 -> [sTmIn_D_u8BexvCalibSts]
  sTmDiag_D_u8BexvFltSt/1 -> [sTmDiag_D_u8BexvFltSt]
  sTmDiag_D_u8EexvFltSt/1 -> [sTmDiag_D_u8EexvFltSt]
  sTmDiag_D_u8CexvFltSt/1 -> [sTmDiag_D_u8CexvFltSt]
  sTmRefriModeMgr_D_u8HpModeCmd/1 -> [sTmRefriModeMgr_D_u8HpModeCmd]
  sTmSigProces_Te_s32TempInlet/1 -> [sTmSigProces_Te_s32TempInlet]
  sTmSigProces_Te_s32CurOutSC/1 -> [sTmSigProces_Te_s32CurOutSC]
  yTmRefriModeMgr_B_CoolModeInCycle/1 -> [yTmRefriModeMgr_B_CoolModeInCycle]
  sTmSigProces_Te_s32HvBattCooltTFilter/1 -> [sTmSigProces_Te_s32HvBattCooltTFilter]
  sTmRefriModeMgr_D_u8HPCurMode/1 -> [sTmRefriModeMgr_D_u8HPCurMode]
  sTmRefriModeMgr_D_u8HpModeMainState/1 -> [sTmRefriModeMgr_D_u8HpModeMainState]
  sTmSigProces_Te_s32CurSCCalValue/1 -> [sTmSigProces_Te_s32CurSCCalValue]
  yTmRefriModeMgr_B_InterChillDeicing/1 -> [yTmRefriModeMgr_B_InterChillDeicing]
  sTmSigProces_Te_s32HvBattCooltTOutFilter/1 -> [sTmSigProces_Te_s32HvBattCooltTOutFilter]
  sTmSigProces_Te_s32TAmb/1 -> [sTmSigProces_Te_s32TAmb]
  sTmSigProces_D_u8CarChrgMode/1 -> [sTmSigProces_D_u8CarChrgMode]
  sTmIn_D_u8HvBattCoolgReq/1 -> [sTmIn_D_u8HvBattCoolgReq]
  sTmIn_Te_s32HvBattCooltTReq/1 -> [sTmIn_Te_s32HvBattCooltTReq]
  sTmSigProces_Te_s32HeatSH/1 -> [sTmSigProces_Te_s32HeatSH]
  yTmRefriModeMgr_B_CoolOCRMode/1 -> [yTmRefriModeMgr_B_CoolOCRMode]
  sTmSigProces_Te_s32EvapFanReqRamp/1 -> [sTmSigProces_Te_s32EvapFanReqRamp]
  sTmIn_v_s32VehSpdLgt/1 -> [sTmIn_v_s32VehSpdLgt]
  sTmSigProces_Te_s32BattHvMaxFilter/1 -> [sTmSigProces_Te_s32BattHvMaxFilter]
  sTmSigProces_Te_s32EvapFanFilter/1 -> [sTmSigProces_Te_s32EvapFanFilter]
  sTmComprCtrl_n_u16CompRpmReq/1 -> [sTmComprCtrl_n_u16CompRpmReq]
  sTmComprCtrl_n_u16CompMaxRpm/1 -> [sTmComprCtrl_n_u16CompMaxRpm]
  sTmSigProces_Te_s32HeatrAirTReqRamp/1 -> [sTmSigProces_Te_s32HeatrAirTReqRamp]
  sTmSigProces_md_u16BlwHeat/1 -> [sTmSigProces_md_u16BlwHeat]
  sTmSigProces_p_u16PHighSide/1 -> [sTmSigProces_p_u16PHighSide]
  sTmSigProces_Te_s32CompDischarge/1 -> [sTmSigProces_Te_s32CompDischarge]
  yTmIn_B_HmiMaxACReq/1 -> [yTmIn_B_HmiMaxACReq]
  sTmSigProces_Te_s32InletCal/1 -> [sTmSigProces_Te_s32InletCal]
  sTmSigProces_Te_s32CoolSH/1 -> [sTmSigProces_Te_s32CoolSH]
  sTmSigProces_p_u16PLowSide/1 -> [sTmSigProces_p_u16PLowSide]
  sTmSigProces_md_u16BlwCool/1 -> [sTmSigProces_md_u16BlwCool]
  sTmSigProces_Te_s32CurInterSC/1 -> [sTmSigProces_Te_s32CurInterSC]
  yTmHvchCtrl_B_HpcPtcEnad/1 -> [yTmHvchCtrl_B_HpcPtcEnad]
  sTmRefriModeMgr_D_u8HpReqPTCState/1 -> [sTmRefriModeMgr_D_u8HpReqPTCState]
  yTmComprCtrl_B_CompOnReq/1 -> [yTmComprCtrl_B_CompOnReq]
  sTmIn_D_u8HeatPump/1 -> [sTmIn_D_u8HeatPump]
  sTmSigProces_Te_s32HvacHexAirTFilter/1 -> [sTmSigProces_Te_s32HvacHexAirTFilter]
  sTmDiag_D_u8EexvPosnReq2FEnaState/1 -> [sTmDiag_D_u8EexvPosnReq2FEnaState]
  sTmDiag_X_s32EexvPosnReq2F/1 -> [sTmDiag_X_s32EexvPosnReq2F]
  sTmDiag_D_u8EexvMoveEna2FEnaState/1 -> [sTmDiag_D_u8EexvMoveEna2FEnaState]
  yTmDiag_B_EexvMoveEnReq2F/1 -> [yTmDiag_B_EexvMoveEnReq2F]
  sTmDiag_D_u8EexvCal2FEnaState/1 -> [sTmDiag_D_u8EexvCal2FEnaState]
  yTmDiag_B_EexvCalReq2F/1 -> [yTmDiag_B_EexvCalReq2F]
  sTmDiag_D_u8BexvPosnReq2FEnaState/1 -> [sTmDiag_D_u8BexvPosnReq2FEnaState]
  sTmDiag_X_s32BexvPosnReq2F/1 -> [sTmDiag_X_s32BexvPosnReq2F]
  sTmDiag_D_u8BexvMoveEna2FEnaState/1 -> [sTmDiag_D_u8BexvMoveEna2FEnaState]
  yTmDiag_B_BexvMoveEnReq2F/1 -> [yTmDiag_B_BexvMoveEnReq2F]
  sTmDiag_D_u8BexvCal2FEnaState/1 -> [sTmDiag_D_u8BexvCal2FEnaState]
  yTmDiag_B_BexvCalReq2F/1 -> [yTmDiag_B_BexvCalReq2F]
  sTmDiag_D_u8CexvPosnReq2FEnaState/1 -> [sTmDiag_D_u8CexvPosnReq2FEnaState]
  sTmDiag_X_s32CexvPosnReq2F/1 -> [sTmDiag_X_s32CexvPosnReq2F]
  sTmDiag_D_u8CexvMoveEna2FEnaState/1 -> [sTmDiag_D_u8CexvMoveEna2FEnaState]
  yTmDiag_B_CexvMoveEnReq2F/1 -> [yTmDiag_B_CexvMoveEnReq2F]
  sTmDiag_D_u8CexvCal2FEnaState/1 -> [sTmDiag_D_u8CexvCal2FEnaState]
  yTmDiag_B_CexvCalReq2F/1 -> [yTmDiag_B_CexvCalReq2F]
  sTmSigProces_D_u8LargerCoolingFlag/1 -> [sTmSigProces_D_u8LargerCoolingFlag]
  sTmComprCtrl_D_u8HvacFlowLevel/1 -> [sTmComprCtrl_D_u8HvacFlowLevel]
  sTmRefriModeMgr_D_u8ModeSwitchType/1 -> [sTmRefriModeMgr_D_u8ModeSwitchType]
  sTmComprCtrl_D_u8CmprRefriSwitchSt/1 -> [sTmComprCtrl_D_u8CmprRefriSwitchSt]
  sTmIn_X_s32EexvPosSts/1 -> [sTmIn_X_s32EexvPosSts]
  sTmIn_X_s32CexvPosSts/1 -> [sTmIn_X_s32CexvPosSts]
  sTmIn_X_s32BexvPosSts/1 -> [sTmIn_X_s32BexvPosSts]
  sTmSovCtrl_D_u8SOV2RefriSwitchSt/1 -> [sTmSovCtrl_D_u8SOV2RefriSwitchSt]
  sTmDiag_D_u8EvapOutTFltSt/1 -> [sTmDiag_D_u8EvapOutTFltSt]
  sTmDiag_D_u8ChillerOutTFltSt/1 -> [sTmDiag_D_u8ChillerOutTFltSt]
  sTmDiag_D_u8LoSidePFltSt/1 -> [sTmDiag_D_u8LoSidePFltSt]
  sTmDiag_D_u8HiSidePFltSt/1 -> [sTmDiag_D_u8HiSidePFltSt]
  sTmDiag_D_u8OutrCondOutTFltSt/1 -> [sTmDiag_D_u8OutrCondOutTFltSt]
  sTmDiag_D_u8InrCondOutTFltSt/1 -> [sTmDiag_D_u8InrCondOutTFltSt]
  sTmSigProces_Pw_i16ReqPwrForCool/1 -> [sTmSigProces_Pw_i16ReqPwrForCool]
  sTmIn_L_s32HvBattCoolFlow1/1 -> [sTmIn_L_s32HvBattCoolFlow1]
  [sTmRefriVlvCtrl_X_s32CEXVPosReq] -> rAfter2_X_s32CEXVPosReq/1
  [sTmRefriVlvCtrl_X_s32EEXVPosReq] -> rAfter2_X_s32EEXVPosReq/1
  [sTmRefriVlvCtrl_X_s32BEXVPosReq] -> rAfter2_X_s32BEXVPosReq/1
  [yTmRefriVlvCtrl_B_HpcCexvMovEnable] -> xAfter2_B_HpcCexvMovEnable/1
  [sTmRefriVlvCtrl_Z_u8CEXVInitState] -> rAfter2_Z_u8CEXVInitState/1
  [yTmRefriVlvCtrl_B_CexvCalibReq] -> xAfter2_B_CexvCalibReq/1
  [yTmRefriVlvCtrl_B_HpcEexvMovEnable] -> xAfter2_B_HpcEexvMovEnable/1
  [sTmRefriVlvCtrl_Z_u8EEXVInitState] -> rAfter2_Z_u8EEXVInitState/1
  [yTmRefriVlvCtrl_B_EexvCalibReq] -> xAfter2_B_EexvCalibReq/1
  [yTmRefriVlvCtrl_B_HpcBexvMovEnable] -> xAfter2_B_HpcBexvMovEnable/1
  [sTmRefriVlvCtrl_Z_u8BEXVInitState] -> rAfter2_Z_u8BEXVInitState/1
  [yTmRefriVlvCtrl_B_BexvCalibReq] -> xAfter2_B_BexvCalibReq/1
  [sTmRefriVlvCtrl_X_s32SM3BexvMaxPos] -> rAfter2_X_s32SM3BexvMaxPos/1
  [yTmRefriVlvCtrl_B_EvapBattTLimBexvEna] -> xAfter2_B_EvapBattTLimBexvEna/1
  [sTmRefriVlvCtrl_D_u8EexvRefriSwitchSt] -> rAfter2_D_u8EexvRefriSwitchSt/1
  [sTmRefriVlvCtrl_D_u8CexvRefriSwitchSt] -> rAfter2_D_u8CexvRefriSwitchSt/1
  [sTmRefriVlvCtrl_D_u8BexvRefriSwitchSt] -> rAfter2_D_u8BexvRefriSwitchSt/1
